simulink model "rtdemo1"  (Simulink 7.7)
settings: Solver=ode4  StartTime=0.0  StopTime=inf  FixedStep=0.001  RelTol=1e-3
libraries: opal_lib x4, rtlab x2, simulink x1
Description:
  | Model of a simple control system for use iin training.
settings Model: Creator=Paul Baracos  LastModifiedBy=DanielOBrien
settings DataIOCC: SaveOutput=off  SaveTime=off  SignalLoggingName=sigsOut
settings OptimizationCC: BlockReduction=off  BooleanDataType=off  OptimizeBlockIOStorage=off  BufferReuse=off  ExpressionFolding=off  LocalBlockOutputs=off  InitFltsAndDblsToZero=on
settings DebuggingCC: SaveWithParameterizedLinksMsg=none  SignalResolutionControl=TryResolveAllWithWarning  SolverPrmCheckMsg=none  MultiTaskDSMMsg=warning  MultiTaskCondExecSysMsg=none  FcnCallInpInsideContextMsg=Enable All  StrictBusMsg=None
settings HardwareCC: TargetUnknown=on
settings CodeAppCC: CustomSymbolStrType=$N$R$M_T
settings GRTTargetCC: TargetFcnLib=ansi_tfl_tmw.mat  TargetFunctionLibrary=C89/C90 (ANSI)

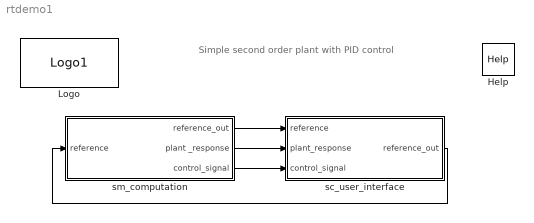
== system rtdemo1 ==
  note: Simple second order plant with PID control
  Help : opal_lib/Help  docfile=../help/help.html
  Logo : opal_lib/Logo1  vide=[]
  sc_user_interface : Subsystem
  sm_computation : Subsystem
  wires:
  sc_user_interface/1(reference_out) -> sm_computation/1(reference)
  sm_computation/3(control_signal) -> sc_user_interface/3(control_signal)
  sm_computation/2(plant _response) -> sc_user_interface/2(plant_response)
  sm_computation/1(reference_out) -> sc_user_interface/1(reference)

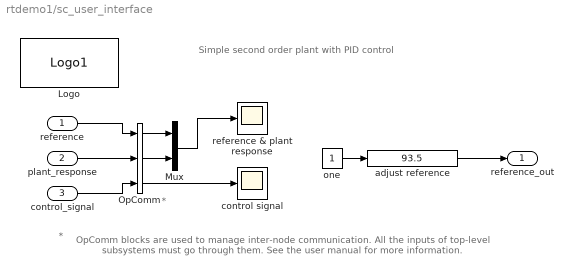
== system rtdemo1/sc_user_interface ==
  note: Simple second order plant with PID control
  note: OpComm blocks are used to manage inter-node communication. All the inputs of top-level
      | subsystems must go through them. See the user manual for more information.
  note: *
  note: *
  reference : Inport
  plant_response : Inport  Port=2
  control_signal : Inport  Port=3
  Logo : opal_lib/Logo1  vide=[]
  Mux : Mux  Inputs=2
  OpComm : rtlab/OpComm  nbport=3  groupe_acq=1  subsys_rate=0  st=0  Synchronization=on  Interpolation=on  Threshold=1.0  Missed_Data=off  Sim_Time=off  Samples=off  dynSigOut=off  from_console=0  warning_done=off  writeOpCommFile=off  Offset=off
  adjust reference : simulink/Math Operations/Slider Gain  low=0  gain=93.5  high=100
  control signal : Scope
      settings: YMin=-200  YMax=200  SaveName=controlSignal
  one : Constant
  reference & plant response : Scope
      settings: Tag=op_tm_save_it  TimeRange=10  YMin=0  YMax=160  SaveName=referenceAndPlant
  reference_out : Outport
  wires:
  Mux/1 -> reference & plant response/1
  reference/1 -> OpComm/1
  control_signal/1 -> OpComm/3
  plant_response/1 -> OpComm/2
  OpComm/1 -> Mux/1
  OpComm/2 -> Mux/2
  OpComm/3 -> control signal/1
  adjust reference/1 -> reference_out/1
  one/1 -> adjust reference/1

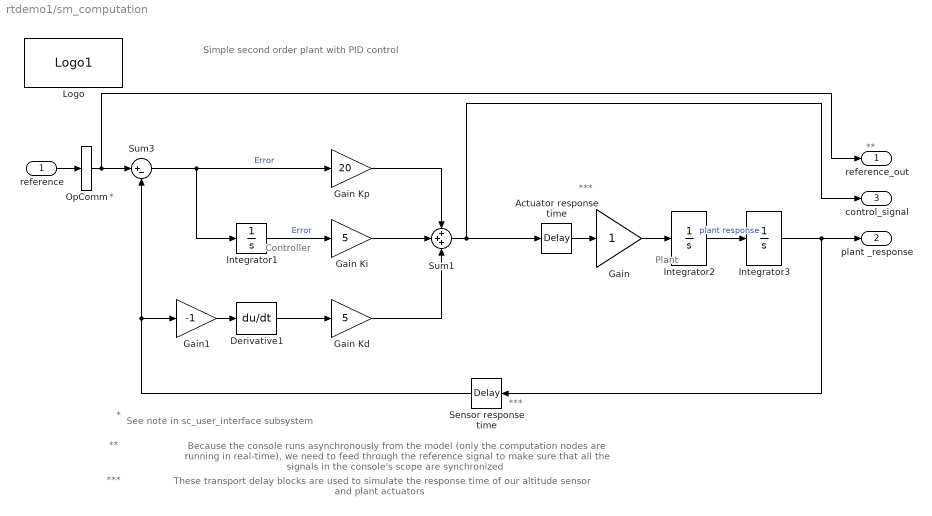
== system rtdemo1/sm_computation ==
  note: Controller
  note: Plant
  note: Simple second order plant with PID control
  note: Because the console runs asynchronously from the model (only the computation nodes are running in real-time), we
      | need to feed through the reference signal to make sure that all the signals in the console's scope are synchronized
  note: **
  note: **
  note: *
  note: See note in sc_user_interface subsystem
  note: *
  note: ***
  note: These transport delay blocks are used to simulate the response time of our altitude sensor and plant actuators
  note: ***
  note: ***
  reference : Inport
  Actuator response time : TransportDelay  DelayTime=0.005  BufferSize=1+ceil(0.005/eval(get_param(bdroot, 'FixedStep')))
  Derivative1 : Derivative
  Gain : Gain  SaturateOnIntegerOverflow=on  OutDataTypeStr=Inherit: Same as input  ParamDataTypeStr=Inherit: Same as input
  Gain Kd : Gain  Gain=5  SaturateOnIntegerOverflow=on  OutDataTypeStr=Inherit: Same as input  ParamDataTypeStr=Inherit: Same as input
  Gain Ki : Gain  Gain=5  SaturateOnIntegerOverflow=on  OutDataTypeStr=Inherit: Same as input  ParamDataTypeStr=Inherit: Same as input
  Gain Kp : Gain  Gain=20  SaturateOnIntegerOverflow=on  OutDataTypeStr=Inherit: Same as input  ParamDataTypeStr=Inherit: Same as input
  Gain1 : Gain  Gain=-1  SaturateOnIntegerOverflow=on  OutDataTypeStr=Inherit: Same as input  ParamDataTypeStr=Inherit: Same as input
  Integrator1 : Integrator
  Integrator2 : Integrator
  Integrator3 : Integrator  LimitOutput=on  UpperSaturationLimit=200  LowerSaturationLimit=0
  Logo : opal_lib/Logo1  vide=[]
  OpComm : rtlab/OpComm  nbport=1  groupe_acq=1  subsys_rate=0  st=0  Synchronization=on  Interpolation=on  Threshold=1.0  Missed_Data=off  Sim_Time=off  Samples=off  dynSigOut=off  from_console=0  warning_done=off  writeOpCommFile=off  Offset=off
  Sensor response time : TransportDelay  DelayTime=0.005  BufferSize=1+ceil(0.005/eval(get_param(bdroot, 'FixedStep')))
  Sum1 : Sum  Inputs=+++  SaturateOnIntegerOverflow=on  InputSameDT=on  OutDataTypeStr=Inherit: Same as first input
  Sum3 : Sum  Inputs=|+-  SaturateOnIntegerOverflow=on  InputSameDT=on  OutDataTypeStr=Inherit: Same as first input
  reference_out : Outport
  plant _response : Outport  Port=2
  control_signal : Outport  Port=3
  wires:
  reference/1 -> OpComm/1
  OpComm/1 -> Sum3/1, reference_out/1
  Sum3/1 -> Gain Kp/1, Integrator1/1  "Error"
  Gain Kp/1 -> Sum1/1
  Integrator1/1 -> Gain Ki/1  "Error"
  Derivative1/1 -> Gain Kd/1
  Gain Ki/1 -> Sum1/2
  Gain1/1 -> Derivative1/1
  Gain Kd/1 -> Sum1/3
  Sum1/1 -> control_signal/1, Actuator response time/1
  Sensor response time/1 -> Sum3/2, Gain1/1
  Integrator2/1 -> Integrator3/1  "plant response"
  Integrator3/1 -> plant _response/1, Sensor response time/1
  Gain/1 -> Integrator2/1
  Actuator response time/1 -> Gain/1
